simulink model "TASK_21"  (R2018b)
settings: Solver=VariableStepAuto  StartTime=0.0  StopTime=100  RelTol=1e-3
libraries: simulink x2, simulink_extras x1
settings Model: Creator=Федор  LastModifiedBy=Федор

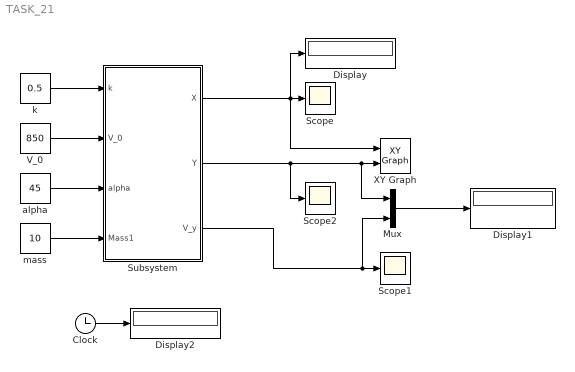
== system TASK_21 ==
  Clock : Clock
  Display : Display
  Display1 : Display
  Display2 : Display
  Mux : Mux  Inputs=2
  Scope : Scope
  Scope1 : Scope
  Scope2 : Scope
  Subsystem : Subsystem
  V_0 : Constant  Value=850
  XY Graph : simulink/Sinks/XY Graph  xmin=0  xmax=10000  ymin=0  ymax=10000  st=-1
  alpha : Constant  Value=45
  k : Constant  Value=0.5
  mass : Constant  Value=10
  wires:
  mass/1 -> Subsystem/4(Mass1)
  alpha/1 -> Subsystem/3(alpha)
  V_0/1 -> Subsystem/2(V_0)
  k/1 -> Subsystem/1(k)
  Subsystem/2(Y) -> Scope2/1, Mux/1, XY Graph/2
  Subsystem/1(X) -> Display/1, Scope/1, XY Graph/1
  Subsystem/3(V_y) -> Mux/2, Scope1/1
  Mux/1 -> Display1/1
  Clock/1 -> Display2/1

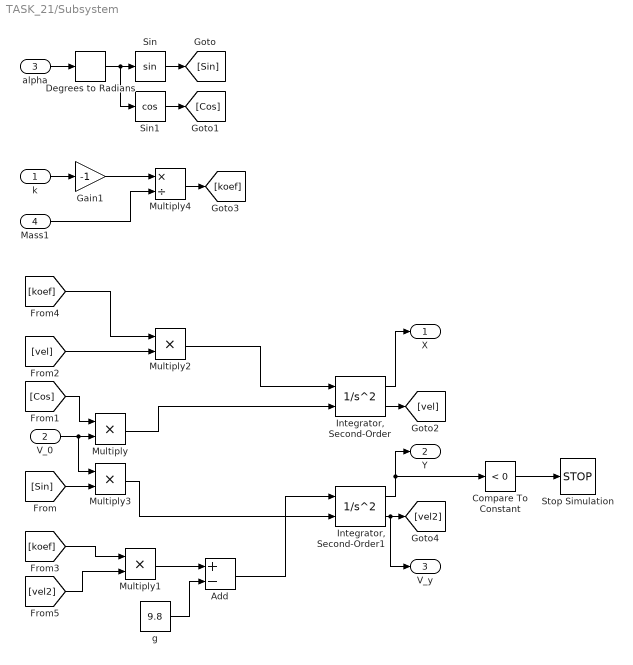
== system TASK_21/Subsystem ==
  k : Inport
  V_0 : Inport  Port=2
  alpha : Inport  Port=3
  Mass1 : Inport  Port=4
  Add : Sum  Inputs=+-
  Compare To Constant : simulink/Logic and Bit Operations/Compare To Constant  relop=<  const=0  OutDataTypeStr=boolean
  Degrees to Radians : simulink_extras/Transformations/Degrees to Radians
  Gain1 : Gain  Gain=-1
  "Integrator, Second-Order" : SecondOrderIntegrator  ICSourceDXDT=external
  "Integrator, Second-Order1" : SecondOrderIntegrator  ICSourceDXDT=external
  Multiply{,1..3} (4 alike) : Product
  Multiply4 : Product  Inputs=*/
  Sin : Trigonometry
  Sin1 : Trigonometry  Operator=cos
  Stop Simulation : Stop
  g : Constant  Value=9.8
  X : Outport
  Y : Outport  Port=2
  V_y : Outport  Port=3
  wires:
  alpha/1 -> Degrees to Radians/1
  Degrees to Radians/1 -> Sin1/1, Sin/1
  Sin/1 -> [Sin]
  Sin1/1 -> [Cos]
  "Integrator, Second-Order"/1 -> X/1
  "Integrator, Second-Order"/2 -> [vel]
  Multiply/1 -> "Integrator, Second-Order"/2
  [koef] -> Multiply2/1
  [vel] -> Multiply2/2
  Multiply2/1 -> "Integrator, Second-Order"/1
  V_0/1 -> Multiply3/1, Multiply/2
  [Cos] -> Multiply/1
  [Sin] -> Multiply3/2
  k/1 -> Gain1/1
  Gain1/1 -> Multiply4/1
  Mass1/1 -> Multiply4/2
  Multiply4/1 -> [koef]
  Multiply3/1 -> "Integrator, Second-Order1"/2
  "Integrator, Second-Order1"/2 -> V_y/1, [vel2]
  [koef] -> Multiply1/1
  [vel2] -> Multiply1/2
  "Integrator, Second-Order1"/1 -> Compare To Constant/1, Y/1
  g/1 -> Add/2
  Multiply1/1 -> Add/1
  Add/1 -> "Integrator, Second-Order1"/1
  Compare To Constant/1 -> Stop Simulation/1
